simulink model "model_no_linear1"  (R2022a)
settings: Solver=VariableStepAuto  StartTime=0  StopTime=200  RelTol=1e-3
values from neighbouring files (symbols this model uses):
  amplitude_entrada = 1    [ball_and_beam_pfc.m]
  bool_degrau = 1    [ball_and_beam_pfc.m]
  C = [0 0 1 0]    [ball_and_beam_pfc.m]
  g = 9.8    [ball_and_beam_pfc.m]    (also in nonlinear_ball_and_beam.m)
  Jv = (1/2) * mv * L^2    (= 0.058703125)    [ball_and_beam_pfc.m]    (also in nonlinear_ball_and_beam.m)
  L = 0.425    [ball_and_beam_pfc.m]    (also in nonlinear_ball_and_beam.m)
  mb = 0.064    [ball_and_beam_pfc.m]    (also in nonlinear_ball_and_beam.m)
  mv = 0.65    [ball_and_beam_pfc.m]    (also in nonlinear_ball_and_beam.m)
undefined symbols (not defined in the file or in its folder): k_seguimento, ki_seguimento
settings Model: Creator=Notebook_Artur  LastModifiedBy=Notebook_Artur

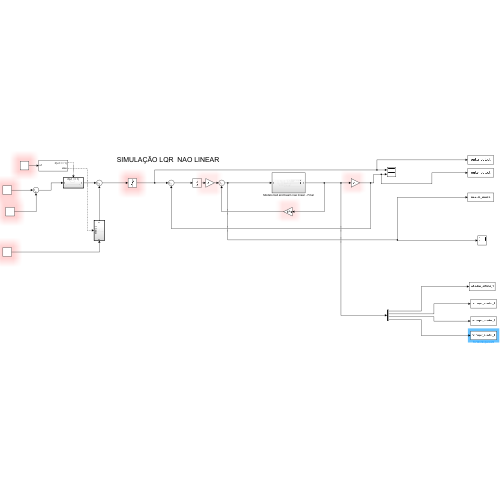
[thumbnail: Simulink's stored preview of the top-level diagram]
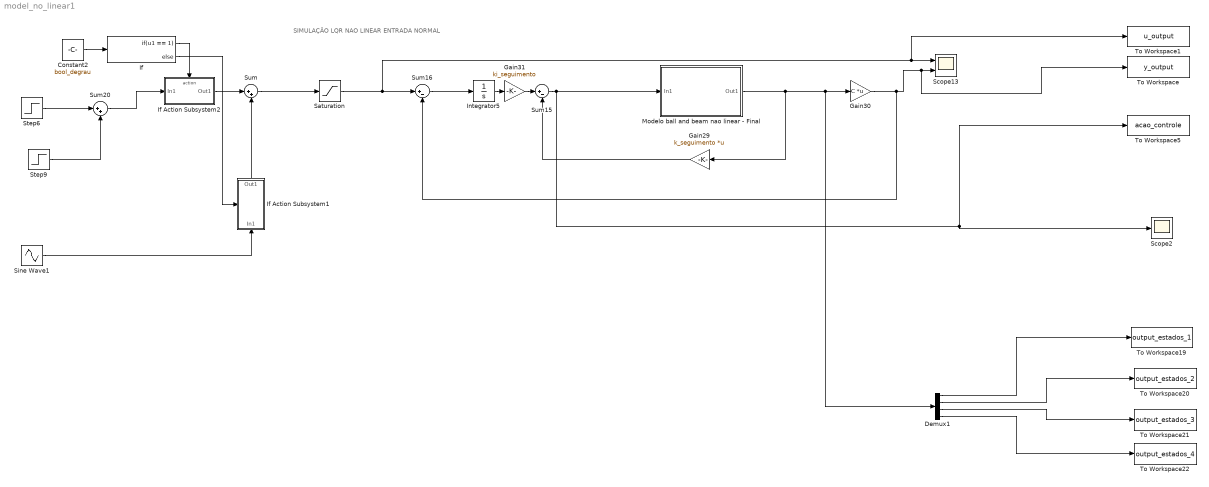
== system model_no_linear1 ==
  note: SIMULAÇÃO LQR NAO LINEAR ENTRADA NORMAL
  Constant2 : Constant  Value=bool_degrau
  Demux1 : Demux
  Gain29 : Gain  Gain=k_seguimento  Multiplication=Matrix(K*u)
  Gain30 : Gain  Gain=C  Multiplication=Matrix(K*u)
  Gain31 : Gain  Gain=ki_seguimento
  If : If  IfExpression=u1 == 1
  If Action Subsystem1 : Subsystem  TreatAsAtomicUnit=on
  If Action Subsystem2 : Subsystem  TreatAsAtomicUnit=on
  Integrator5 : Integrator
  Modelo ball and beam nao linear - Final : Subsystem
  Saturation : Saturate  UpperLimit=L/2  LowerLimit=-L/2
  Scope13 : Scope  NumInputPorts=2
  Scope2 : Scope
  Sine Wave1 : Sin  Amplitude=amplitude_entrada  Frequency=0.1  SampleTime=0
  Step6 : Step  After=amplitude_entrada  SampleTime=0
  Step9 : Step  Time=100  After=-2*amplitude_entrada  SampleTime=0
  Sum : Sum  Inputs=|++
  Sum15 : Sum  Inputs=|+-
  Sum16 : Sum  Inputs=|+-
  Sum20 : Sum  Inputs=|++
  To Workspace : ToWorkspace  VariableName=y_output  SaveFormat=Timeseries  SampleTime=-1
  To Workspace1 : ToWorkspace  VariableName=u_output  SaveFormat=Timeseries  SampleTime=-1
  To Workspace19 : ToWorkspace  VariableName=output_estados_1  SaveFormat=Timeseries  SampleTime=-1
  To Workspace20 : ToWorkspace  VariableName=output_estados_2  SaveFormat=Timeseries  SampleTime=-1
  To Workspace21 : ToWorkspace  VariableName=output_estados_3  SaveFormat=Timeseries  SampleTime=-1
  To Workspace22 : ToWorkspace  VariableName=output_estados_4  SaveFormat=Timeseries  SampleTime=-1
  To Workspace5 : ToWorkspace  VariableName=acao_controle  SaveFormat=Timeseries  SampleTime=-1
  wires:
  Integrator5/1 -> Gain31/1
  Demux1/1 -> To Workspace19/1
  Gain31/1 -> Sum15/1
  Modelo ball and beam nao linear - Final/1(Out1) -> Demux1/1, Gain30/1, Gain29/1
  Step9/1 -> Sum20/2
  Demux1/4 -> To Workspace22/1
  Sum15/1 -> Modelo ball and beam nao linear - Final/1(In1), To Workspace5/1, Scope2/1
  Sum16/1 -> Integrator5/1
  Sum/1 -> Saturation/1
  If/1 -> If Action Subsystem2/Action
  Demux1/2 -> To Workspace20/1
  Sum20/1 -> If Action Subsystem2/1(In1)
  If Action Subsystem1/1(Out1) -> Sum/2
  If/2 -> If Action Subsystem1/Action
  Step6/1 -> Sum20/1
  Saturation/1 -> To Workspace1/1, Scope13/1, Sum16/1
  If Action Subsystem2/1(Out1) -> Sum/1
  Gain29/1 -> Sum15/2
  Demux1/3 -> To Workspace21/1
  Constant2/1 -> If/1
  Gain30/1 -> Sum16/2, To Workspace/1, Scope13/2
  Sine Wave1/1 -> If Action Subsystem1/1(In1)

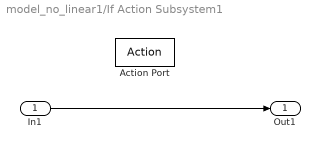
== system model_no_linear1/If Action Subsystem1 ==
  In1 : Inport
  Action Port : ActionPort  ActionPortLabel=else
  Out1 : Outport
  wires:
  In1/1 -> Out1/1

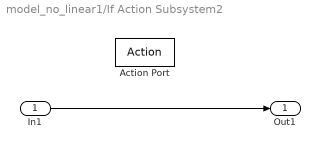
== system model_no_linear1/If Action Subsystem2 ==
  In1 : Inport
  Action Port : ActionPort  ActionPortLabel=if(u1 == 1)
  Out1 : Outport
  wires:
  In1/1 -> Out1/1

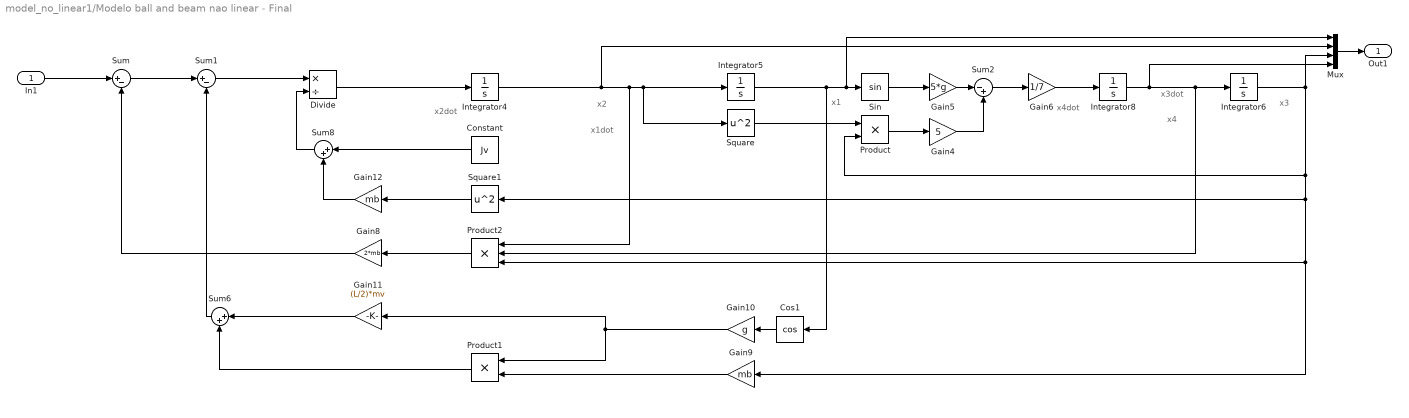
== system model_no_linear1/Modelo ball and beam nao linear - Final ==
  note: x3
  note: x3dot
  note: x4
  note: x4dot
  note: x1
  note: x1dot
  note: x2dot
  note: x2
  In1 : Inport
  Constant : Constant  Value=Jv
  Cos1 : Trigonometry  Operator=cos
  Divide : Product  Inputs=*/
  Gain10 : Gain  Gain=g
  Gain11 : Gain  Gain=(L/2)*mv
  Gain12 : Gain  Gain=mb
  Gain4 : Gain  Gain=5
  Gain5 : Gain  Gain=5*g
  Gain6 : Gain  Gain=1/7
  Gain8 : Gain  Gain=2*mb
  Gain9 : Gain  Gain=mb
  Integrator{4..6,8} (4 alike) : Integrator
  Mux : Mux
  Product : Product
  Product1 : Product
  Product2 : Product  Inputs=3
  Sin : Trigonometry
  Square : Math  Operator=square
  Square1 : Math  Operator=square
  Sum : Sum  Inputs=|+-
  Sum1 : Sum  Inputs=|+-
  Sum2 : Sum  Inputs=|-+
  Sum6 : Sum  Inputs=|++
  Sum8 : Sum  Inputs=|++
  Out1 : Outport
  wires:
  Integrator8/1 -> Mux/4, Product2/2, Integrator6/1
  Integrator5/1 -> Cos1/1, Mux/1, Sin/1
  Sum6/1 -> Sum1/2
  Sum2/1 -> Gain6/1
  Gain10/1 -> Product1/1, Gain11/1
  Square/1 -> Product/1
  Integrator6/1 -> Mux/3, Gain9/1, Product2/3, Square1/1, Product/2
  Gain11/1 -> Sum6/1
  Gain12/1 -> Sum8/2
  Gain6/1 -> Integrator8/1
  Gain4/1 -> Sum2/2
  Gain9/1 -> Product1/2
  Cos1/1 -> Gain10/1
  Divide/1 -> Integrator4/1
  Product2/1 -> Gain8/1
  Product/1 -> Gain4/1
  Square1/1 -> Gain12/1
  Sum8/1 -> Divide/2
  Product1/1 -> Sum6/2
  Constant/1 -> Sum8/1
  Mux/1 -> Out1/1
  Gain5/1 -> Sum2/1
  Sin/1 -> Gain5/1
  Gain8/1 -> Sum/2
  Sum1/1 -> Divide/1
  Sum/1 -> Sum1/1
  Integrator4/1 -> Mux/2, Product2/1, Square/1, Integrator5/1
  In1/1 -> Sum/1
